simulink model "Pedal_Interpretation_exe"  (Simulink 7.0)
settings: Solver=ode4  StartTime=0.0  StopTime=88  FixedStep=0.01  RelTol=1e-3
InitFcn:
  | PedalInterp_para
values from neighbouring files (symbols this model uses):
  ped_min = 5    [PedalInterp_para.m]
  T_max_Brake = 4000    [PedalInterp_para.m]
  TI = 0    [PAS_callback.m]
undefined symbols (not defined in the file or in its folder): fzgbib, m_ab_100pro, m_ab_70pro, PedalInterpretation, v_bereich
libraries: simulink x320
(part 23 of 23)

== system Pedal_Interpretation_exe/Validation Functions/SR-PI-02.2 Acceleration pedal interpretation/T_des_Drive increases /PAS/none - pass - fail/Compute delay1/Hold1 ==
  " " : Inport  OutDataType=sfix(16)  OutScaling=2^0
  "    " : Inport  Port=2  OutDataType=sfix(16)  OutScaling=2^0
  Memory : Memory  Orientation=left
  Switch : Switch  Criteria=u2 ~= 0
  "  " : Outport  OutDataType=sfix(16)  OutScaling=2^0
  wires:
  Memory/1 -> Switch/3
  Switch/1 -> Memory/1, "  "/1
  "    "/1 -> Switch/1
  " "/1 -> Switch/2

== system Pedal_Interpretation_exe/Validation Functions/SR-PI-02.2 Acceleration pedal interpretation/T_des_Drive increases /PAS/none - pass - fail/Compute delay2/Hold1 ==
  " " : Inport  OutDataType=sfix(16)  OutScaling=2^0
  "    " : Inport  Port=2  OutDataType=sfix(16)  OutScaling=2^0
  Memory : Memory  Orientation=left
  Switch : Switch  Criteria=u2 ~= 0
  "  " : Outport  OutDataType=sfix(16)  OutScaling=2^0
  wires:
  " "/1 -> Switch/2
  "    "/1 -> Switch/1
  Switch/1 -> "  "/1, Memory/1
  Memory/1 -> Switch/3

== stateflow chart TestData 1/SR-PI-01.1 Brake Pedal recognition/Sequencing of test data in time due to Preconditions ==
  state Precondition1
    state TDataPre1
      entry: TDPre = 1;
    state Init1
      entry: TDPre = 1;
    state Stabilise1
      entry: TDPre = 1;
    Init1 -> TDataPre1 : after(50, tick)
    TDataPre1 -> Stabilise1 : after(100, tick)
    (default) -> Init1
  state Precondition2
    state Stabilise2
      entry: TDPre = 2;
    state Init2
      entry: TDPre = 2;
    state TDataPre2
      entry: TDPre = 2;
    Init2 -> TDataPre2 : after(50, tick)
    TDataPre2 -> Stabilise2 : after(100, tick)
  state wait
    entry: TDPre = 2;
  Stabilise2 -> wait : after(50, tick)
  Stabilise1 -> Init2 : after(50, tick)
  (default) -> wait
  wait -> Init1
  data: Activate input inherited; TDPre output double

== stateflow chart variant dependent  Test Control1/variant dependent Test Control ==
  state TestCase1
    entry: TestCase = 1;
  state TestCase2
    entry: TestCase = 2;
  state TestCase3
    entry: TestCase = 3;
  state TestCase4
    entry: TestCase = 4;
  (default) -> TestCase1 : {variant=1;}
  TestCase1 -> TestCase2 : after(400, tick)
  TestCase2 -> TestCase3 : after(400, tick)
  TestCase3 -> TestCase4 : after(200, tick)
  TestCase4 -> TestCase1 : after(1200, tick)
      | {variant=variant+1;}
  data: TestCase output double; variant output double

== stateflow chart variant dependent/variant dependent Test Control_1 ==
  state TestCase1
    entry: TestCase = 1;
  state TestCase2
    entry: TestCase = 2;
  state TestCase3
    entry: TestCase = 3;
  state TestCase4
    entry: TestCase = 4;
  (default) -> TestCase1 : {variant=1;}
  TestCase1 -> TestCase2 : after(400, tick)
  TestCase2 -> TestCase3 : after(400, tick)
  TestCase3 -> TestCase4 : after(200, tick)
  TestCase4 -> TestCase1 : after(1200, tick)
      | {variant=variant+1;}
  data: TestCase output double; variant output double

== stateflow chart TestData 1/SR-PI-01.3 Acceleration Pedal recognition/Sequencing of test data in time due to Preconditions ==
  state Precondition1
    state TDataPre1
      entry: TDPre = 1;
    state Init1
      entry: TDPre = 1;
    state Stabilise1
      entry: TDPre = 1;
    Init1 -> TDataPre1 : after(50, tick)
    TDataPre1 -> Stabilise1 : after(100, tick)
    (default) -> Init1
  state Precondition2
    state Stabilise2
      entry: TDPre = 2;
    state Init2
      entry: TDPre = 2;
    state TDataPre2
      entry: TDPre = 2;
    Init2 -> TDataPre2 : after(50, tick)
    TDataPre2 -> Stabilise2 : after(100, tick)
  state wait
    entry: TDPre = 2;
  Stabilise2 -> wait : after(50, tick)
  Stabilise1 -> Init2 : after(50, tick)
  (default) -> wait
  wait -> Init1 : after(400, tick)
  data: Activate input inherited; TDPre output double

== stateflow chart TestData 1/SR-PI-02.1 Brake pedal interpretation/Sequencing of test data in time due to Preconditions ==
  state Precondition1
    state TDataPre1
      entry: TDPre = 1;
    state Init1
      entry: TDPre = 1;
    state Stabilise1
      entry: TDPre = 1;
    Init1 -> TDataPre1 : after(50, tick)
    TDataPre1 -> Stabilise1 : after(100, tick)
    (default) -> Init1
  state stop
    entry: TDPre = 2;
  stop -> Precondition1 : after(800, tick)
  Stabilise1 -> stop : after(50, tick)
  (default) -> stop
  data: Activate input inherited; TDPre output double

== stateflow chart TestData 1/SR-PI-02.2 Acceleration pedal interpretation/Sequencing of test data in time due to Preconditions ==
  state Precondition1
    state TDataPre1
      entry: TDPre = 1;
    state Init1
      entry: TDPre = 1;
    state Stabilise1
      entry: TDPre = 1;
    Init1 -> TDataPre1 : after(50, tick)
    TDataPre1 -> Stabilise1 : after(100, tick)
    (default) -> Init1
  state wait
    entry: TDPre = 7;
  state Precondition2
    state Init2
      entry: TDPre = 2;
    state TDataPre2
      entry: TDPre = 2;
    state Stabilise2
      entry: TDPre = 2;
    Init2 -> (junction 118) : after(50, tick)
    TDataPre2 -> Stabilise2 : after(100, tick)
    (junction 118) -> TDataPre2
  state Precondition3
    state Init3
      entry: TDPre = 3;
    state TDataPre3
      entry: TDPre = 3;
    state Stabilise3
      entry: TDPre = 3;
    Init3 -> (junction 119) : after(50, tick)
    TDataPre3 -> Stabilise3 : after(100, tick)
    (junction 119) -> TDataPre3
  state Precondition4
    state Init4
      entry: TDPre = 4;
    state TDataPre4
      entry: TDPre = 4;
    state Stabilise4
      entry: TDPre = 4;
    Init4 -> (junction 120) : after(50, tick)
    TDataPre4 -> Stabilise4 : after(100, tick)
    (junction 120) -> TDataPre4
  state Precondition5
    state Init5
      entry: TDPre = 5;
    state TDataPre5
      entry: TDPre = 5;
    state Stabilise5
      entry: TDPre = 5;
    Init5 -> TDataPre5 : after(50, tick)
    TDataPre5 -> Stabilise5 : after(100, tick)
  state Precondition6
    state Init6
      entry: TDPre = 6;
    state TDataPre6
      entry: TDPre = 6;
    state Stabilise6
      entry: TDPre = 6;
    Init6 -> TDataPre6 : after(50, tick)
    TDataPre6 -> Stabilise6 : after(100, tick)
  (junction 114) -> Init3
  (junction 115) -> Init4
  wait -> Precondition1 : after(1000, tick)
  Stabilise1 -> (junction 113) : after(50, tick)
  Stabilise2 -> (junction 114) : after(50, tick)
  Stabilise3 -> (junction 115) : after(50, tick)
  (default) -> wait
  (junction 113) -> Init2
  Stabilise4 -> (junction 116) : after(50, tick)
  (junction 116) -> Init5
  Stabilise5 -> (junction 117) : after(50, tick)
  (junction 117) -> Init6
  Stabilise6 -> wait : after(50, tick)
  data: Activate1 input inherited; TDPre output double; Activate2 input inherited; Activate3 input inherited; Activate4 input inherited; Activate5 input inherited; Activate6 input inherited
